simulink model "test2"  (R2022b)
settings: Solver=VariableStepAuto  StartTime=0.0  StopTime=30.0  RelTol=1e-3
undefined symbols (not defined in the file): fdesignblkfcn, gcbh
libraries: dspfdesign x4, vrlib x1
settings Model: Creator=elsibo  LastModifiedBy=ankurkohli007
settings DebuggingCC: UnconnectedInputMsg=warning  UnconnectedOutputMsg=warning  UnconnectedLineMsg=warning
settings ModelReferenceCC: EnableRefExpFcnMdlSchedulingChecks=on
settings RTWCC: DLArmComputeVersion=19.05

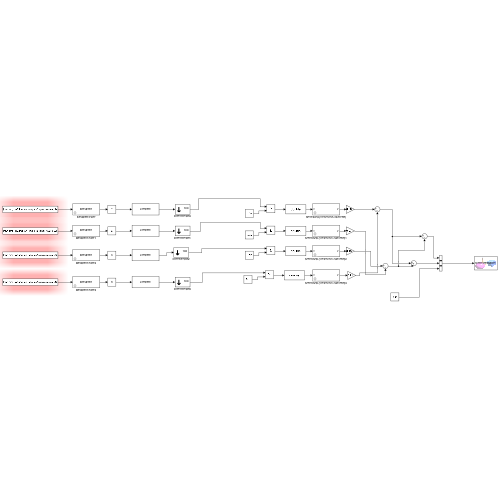
[thumbnail: Simulink's stored preview of the top-level diagram]
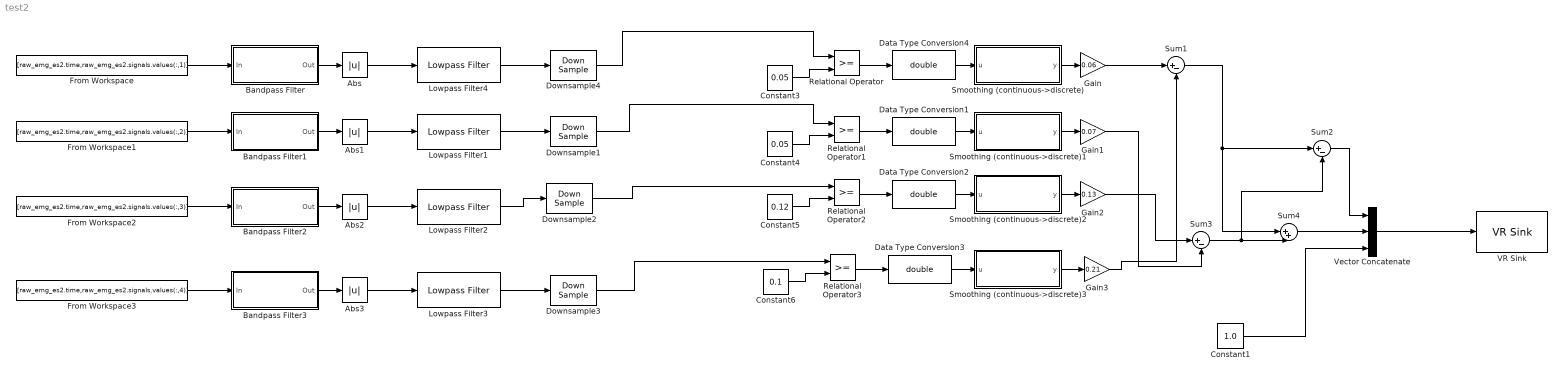
== system test2 ==
  Abs{,1..3} (4 alike) : Abs  SaturateOnIntegerOverflow=off
  Bandpass Filter : Subsystem  DialogController=fdesignblkfcn  InitFcn=fdesignblkfcn(gcbh, {'InitFcn'});  mask(Bandpass Filter){}
      mask help: Design a bandpass filter
      settings: CopyFcn=fdesignblkfcn(gcbh, {'CopyFcn'});
      mask Help: helpview(mapfilelocation('dsp'), 'dspbandpassfilter');
      mask Display: disp('Bandpass');
  Bandpass Filter1 : Subsystem  DialogController=fdesignblkfcn  InitFcn=fdesignblkfcn(gcbh, {'InitFcn'});  mask(Bandpass Filter){}
      mask help: Design a bandpass filter
      settings: CopyFcn=fdesignblkfcn(gcbh, {'CopyFcn'});
      mask Help: helpview(mapfilelocation('dsp'), 'dspbandpassfilter');
      mask Display: disp('Bandpass');
  Bandpass Filter2 : Subsystem  DialogController=fdesignblkfcn  InitFcn=fdesignblkfcn(gcbh, {'InitFcn'});  mask(Bandpass Filter){}
      mask help: Design a bandpass filter
      settings: CopyFcn=fdesignblkfcn(gcbh, {'CopyFcn'});
      mask Help: helpview(mapfilelocation('dsp'), 'dspbandpassfilter');
      mask Display: disp('Bandpass');
  Bandpass Filter3 : Subsystem  DialogController=fdesignblkfcn  InitFcn=fdesignblkfcn(gcbh, {'InitFcn'});  mask(Bandpass Filter){}
      mask help: Design a bandpass filter
      settings: CopyFcn=fdesignblkfcn(gcbh, {'CopyFcn'});
      mask Help: helpview(mapfilelocation('dsp'), 'dspbandpassfilter');
      mask Display: disp('Bandpass');
  Constant1 : Constant  Value=1.0
  Constant3 : Constant  Value=0.05
  Constant4 : Constant  Value=0.05
  Constant5 : Constant  Value=0.12
  Constant6 : Constant  Value=0.1
  Data Type Conversion{1..4} (4 alike) : DataTypeConversion  OutMin=[0.2]  OutMax=[1000]  OutDataTypeStr=double  SaturateOnIntegerOverflow=off  RndMeth=Floor
  Downsample{1..4} (4 alike) : DownSample  N=100  RateOptions=Allow multirate processing
  From Workspace : FromWorkspace  VariableName=[raw_emg_es2.time,raw_emg_es2.signals.values(:,1)]  SampleTime=1/3000
  From Workspace1 : FromWorkspace  VariableName=[raw_emg_es2.time,raw_emg_es2.signals.values(:,2)]  SampleTime=1/3000
  From Workspace2 : FromWorkspace  VariableName=[raw_emg_es2.time,raw_emg_es2.signals.values(:,3)]  SampleTime=1/3000
  From Workspace3 : FromWorkspace  VariableName=[raw_emg_es2.time,raw_emg_es2.signals.values(:,4)]  SampleTime=1/3000
  Gain : Gain  Gain=0.06
  Gain1 : Gain  Gain=0.07
  Gain2 : Gain  Gain=0.13
  Gain3 : Gain  Gain=0.21
  Lowpass Filter{1..4} (4 alike) : dspfdesign/Lowpass Filter  FilterType=FIR  DesignForMinimumOrder=on  FilterOrder=50  PassbandFrequency=3e3  StopbandFrequency=5e3  PassbandRipple=0.1  StopbandAttenuation=80  InheritSampleRate=off  SampleRate=44100  SimulateUsing=Interpreted execution  roundingMode=Floor  coeffsDataTypeStr=fixdt(1,16)
  Relational Operator{,1..3} (4 alike) : RelationalOperator  OutDataTypeStr=boolean  RndMeth=Simplest  InputSameDT=off
  Smoothing (continuous->discrete) : Subsystem  mask(Smoothing (continuous->discrete)){tsSmoothing=0.35, smoothing0=0}
      mask prompts: tsSmoothing "physmod:simscape:couplers:SimscapeNetworkCouplersLib:SmoothingTimeConstants_MP"; smoothing0 "physmod:simscape:couplers:SimscapeNetworkCouplersLib:InitialOutput_MP"
      mask help: physmod:simscape:couplers:SimscapeNetworkCouplersLib:Smoothingcontinuousdiscrete_MD
      mask Help: web([docroot '/physmod/simscape/ref/networkcouplersmoothingcontinuousdiscrete.html'])
  Smoothing (continuous->discrete)1 : Subsystem  mask(Smoothing (continuous->discrete)){tsSmoothing=0.35, smoothing0=0}
      mask prompts: tsSmoothing "physmod:simscape:couplers:SimscapeNetworkCouplersLib:SmoothingTimeConstants_MP"; smoothing0 "physmod:simscape:couplers:SimscapeNetworkCouplersLib:InitialOutput_MP"
      mask help: physmod:simscape:couplers:SimscapeNetworkCouplersLib:Smoothingcontinuousdiscrete_MD
      mask Help: web([docroot '/physmod/simscape/ref/networkcouplersmoothingcontinuousdiscrete.html'])
  Smoothing (continuous->discrete)2 : Subsystem  mask(Smoothing (continuous->discrete)){tsSmoothing=0.35, smoothing0=0}
      mask prompts: tsSmoothing "physmod:simscape:couplers:SimscapeNetworkCouplersLib:SmoothingTimeConstants_MP"; smoothing0 "physmod:simscape:couplers:SimscapeNetworkCouplersLib:InitialOutput_MP"
      mask help: physmod:simscape:couplers:SimscapeNetworkCouplersLib:Smoothingcontinuousdiscrete_MD
      mask Help: web([docroot '/physmod/simscape/ref/networkcouplersmoothingcontinuousdiscrete.html'])
  Smoothing (continuous->discrete)3 : Subsystem  mask(Smoothing (continuous->discrete)){tsSmoothing=0.35, smoothing0=0}
      mask prompts: tsSmoothing "physmod:simscape:couplers:SimscapeNetworkCouplersLib:SmoothingTimeConstants_MP"; smoothing0 "physmod:simscape:couplers:SimscapeNetworkCouplersLib:InitialOutput_MP"
      mask help: physmod:simscape:couplers:SimscapeNetworkCouplersLib:Smoothingcontinuousdiscrete_MD
      mask Help: web([docroot '/physmod/simscape/ref/networkcouplersmoothingcontinuousdiscrete.html'])
  Sum1 : Sum  Inputs=|+-
  Sum2 : Sum  Inputs=|+-
  Sum3 : Sum  Inputs=|+-
  Sum4 : Sum  Inputs=|++
  VR Sink : vrlib/VR Sink  InstantiateOnLoad=on  SampleTime=0.1  ViewEnable=on  RemoteChange=off  RemoteView=off  FieldsWritten=cursor.translation.3.1.1.double  WorldFileName=8_palline_color.wrl  AutoView=off  VideoDimensions=[]  AllowVariableSize=off
  Vector Concatenate : Concatenate  NumInputs=3
  wires:
  From Workspace/1 -> Bandpass Filter/1(In)
  Bandpass Filter/1(Out) -> Abs/1
  Abs/1 -> Lowpass Filter4/1
  Lowpass Filter4/1 -> Downsample4/1
  Abs1/1 -> Lowpass Filter1/1
  Lowpass Filter1/1 -> Downsample1/1
  Bandpass Filter1/1(Out) -> Abs1/1
  From Workspace1/1 -> Bandpass Filter1/1(In)
  Downsample1/1 -> Relational Operator1/1
  Abs2/1 -> Lowpass Filter2/1
  Bandpass Filter2/1(Out) -> Abs2/1
  From Workspace2/1 -> Bandpass Filter2/1(In)
  Downsample2/1 -> Relational Operator2/1
  Abs3/1 -> Lowpass Filter3/1
  Lowpass Filter3/1 -> Downsample3/1
  Bandpass Filter3/1(Out) -> Abs3/1
  From Workspace3/1 -> Bandpass Filter3/1(In)
  Downsample3/1 -> Relational Operator3/1
  Vector Concatenate/1 -> VR Sink/1
  Downsample4/1 -> Relational Operator/1
  Constant3/1 -> Relational Operator/2
  Relational Operator/1 -> Data Type Conversion4/1
  Relational Operator1/1 -> Data Type Conversion1/1
  Constant4/1 -> Relational Operator1/2
  Relational Operator2/1 -> Data Type Conversion2/1
  Constant5/1 -> Relational Operator2/2
  Relational Operator3/1 -> Data Type Conversion3/1
  Constant6/1 -> Relational Operator3/2
  Lowpass Filter2/1 -> Downsample2/1
  Data Type Conversion3/1 -> Smoothing (continuous->discrete)3/1(u)
  Data Type Conversion2/1 -> Smoothing (continuous->discrete)2/1(u)
  Data Type Conversion1/1 -> Smoothing (continuous->discrete)1/1(u)
  Data Type Conversion4/1 -> Smoothing (continuous->discrete)/1(u)
  Smoothing (continuous->discrete)/1(y) -> Gain/1
  Smoothing (continuous->discrete)1/1(y) -> Gain1/1
  Smoothing (continuous->discrete)2/1(y) -> Gain2/1
  Smoothing (continuous->discrete)3/1(y) -> Gain3/1
  Gain/1 -> Sum1/1
  Sum1/1 -> Sum2/1, Sum4/1
  Gain2/1 -> Sum3/1
  Sum3/1 -> Sum4/2, Sum2/2
  Sum4/1 -> Vector Concatenate/2
  Sum2/1 -> Vector Concatenate/1
  Constant1/1 -> Vector Concatenate/3
  Gain3/1 -> Sum1/2
  Gain1/1 -> Sum3/2

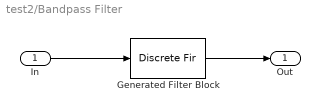
== system test2/Bandpass Filter ==
  In : Inport
  Generated Filter Block : DiscreteFir  Tag=BlockMethodSubSystem  Coefficients=[-0.0867106986736685681 0.172879501957226178 0.0611368344740756825 0.00822498172698654662 -0.0189364689630777752 -0.0305456119635362962 -0.029927052061019966 -0.0224311445482471734 -0.0154422453333472702 -0.0147705811987406625 -0.0205783857487597949 -0.0272517797256104505 -0.0284569945610830509 -0.0221839585574007091 -0.0127406715665240016 -0.00735000555653291324 -0.0102169041814385748 -0.0189181160821402621 -0.0260072397446443268 -0.0250951422264934776 -0.0162958899444141936 -0.00644643769533894805 -0.00372657608997871599 -0.0107951272745376546 -0.0221929620414225356 -0.0284553825598440994 -0.0237986889434766841 -0.0113779247022730377 -0.00119952503274776186 -0.00224663464687881349 -0.0146779403633768464 -0.0289282353463493902 -0.0329178478450258896 -0.0221510441115707439 -0.00434610570060027946 0.00573186727481306366 -0.00179813231379483346 -0.023001586974820111 -0.0413251082228547201 -0.0401288838953623231 -0.0168514574192910466 0.0121051446615590193 0.0218215231144973931 -0.00171807992762008032 -0.0470242140764826691 -0.0802559080529268998 -0.0639028947733619318 0.0153185042045271922 0.13460237441843137 0.241443784310572063 0.283829886850723301 0.241443784310572063 0.13460237441843137 0.0153185042045271922 -0.0639028947733619318 -0.0802559080529268998 -0.0470242140764826691 -0.00171807992762008032 0.0218215231144973931 0.0121051446615590193 -0.0168514574192910466 -0.0401288838953623231 -0.0413251082228547201 -0.023001586974820111 -0.00179813231379483346 0.00573186727481306366 -0.00434610570060027946 -0.0221510441115707439 -0.0329178478450258896 -0.0289282353463493902 -0.0146779403633768464 -0.00224663464687881349 -0.00119952503274776186 -0.0113779247022730377 -0.0237986889434766841 -0.0284553825598440994 -0.0221929620414225356 -0.0107951272745376546 -0.00372657608997871599 -0.00644643769533894805 -0.0162958899444141936 -0.0250951422264934776 -0.0260072397446443268 -0.0189181160821402621 -0.0102169041814385748 -0.00735000555653291324 -0.0127406715665240016 -0.0221839585574007091 -0.0284569945610830509 -0.0272517797256104505 -0.0205783857487597949 -0.0147705811987406625 -0.0154422453333472702 -0.0224311445482471734 -0.029927052061019966 -0.0305456119635362962 -0.0189364689630777752 0.00822498172698654662 0.0611368344740756825 0.172879501957226178 -0.0867106986736685681]  InputProcessing=Columns as channels (frame based)
  Out : Outport  VectorParamsAs1DForOutWhenUnconnected=off
  wires:
  In/1 -> Generated Filter Block/1
  Generated Filter Block/1 -> Out/1

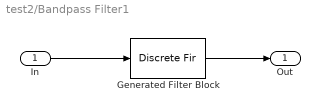
== system test2/Bandpass Filter1 ==
  In : Inport
  Generated Filter Block : DiscreteFir  Tag=BlockMethodSubSystem  Coefficients=[-0.0867106986736685681 0.172879501957226178 0.0611368344740756825 0.00822498172698654662 -0.0189364689630777752 -0.0305456119635362962 -0.029927052061019966 -0.0224311445482471734 -0.0154422453333472702 -0.0147705811987406625 -0.0205783857487597949 -0.0272517797256104505 -0.0284569945610830509 -0.0221839585574007091 -0.0127406715665240016 -0.00735000555653291324 -0.0102169041814385748 -0.0189181160821402621 -0.0260072397446443268 -0.0250951422264934776 -0.0162958899444141936 -0.00644643769533894805 -0.00372657608997871599 -0.0107951272745376546 -0.0221929620414225356 -0.0284553825598440994 -0.0237986889434766841 -0.0113779247022730377 -0.00119952503274776186 -0.00224663464687881349 -0.0146779403633768464 -0.0289282353463493902 -0.0329178478450258896 -0.0221510441115707439 -0.00434610570060027946 0.00573186727481306366 -0.00179813231379483346 -0.023001586974820111 -0.0413251082228547201 -0.0401288838953623231 -0.0168514574192910466 0.0121051446615590193 0.0218215231144973931 -0.00171807992762008032 -0.0470242140764826691 -0.0802559080529268998 -0.0639028947733619318 0.0153185042045271922 0.13460237441843137 0.241443784310572063 0.283829886850723301 0.241443784310572063 0.13460237441843137 0.0153185042045271922 -0.0639028947733619318 -0.0802559080529268998 -0.0470242140764826691 -0.00171807992762008032 0.0218215231144973931 0.0121051446615590193 -0.0168514574192910466 -0.0401288838953623231 -0.0413251082228547201 -0.023001586974820111 -0.00179813231379483346 0.00573186727481306366 -0.00434610570060027946 -0.0221510441115707439 -0.0329178478450258896 -0.0289282353463493902 -0.0146779403633768464 -0.00224663464687881349 -0.00119952503274776186 -0.0113779247022730377 -0.0237986889434766841 -0.0284553825598440994 -0.0221929620414225356 -0.0107951272745376546 -0.00372657608997871599 -0.00644643769533894805 -0.0162958899444141936 -0.0250951422264934776 -0.0260072397446443268 -0.0189181160821402621 -0.0102169041814385748 -0.00735000555653291324 -0.0127406715665240016 -0.0221839585574007091 -0.0284569945610830509 -0.0272517797256104505 -0.0205783857487597949 -0.0147705811987406625 -0.0154422453333472702 -0.0224311445482471734 -0.029927052061019966 -0.0305456119635362962 -0.0189364689630777752 0.00822498172698654662 0.0611368344740756825 0.172879501957226178 -0.0867106986736685681]  InputProcessing=Columns as channels (frame based)
  Out : Outport  VectorParamsAs1DForOutWhenUnconnected=off
  wires:
  In/1 -> Generated Filter Block/1
  Generated Filter Block/1 -> Out/1

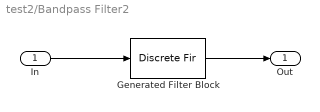
== system test2/Bandpass Filter2 ==
  In : Inport
  Generated Filter Block : DiscreteFir  Tag=BlockMethodSubSystem  Coefficients=[-0.0867106986736685681 0.172879501957226178 0.0611368344740756825 0.00822498172698654662 -0.0189364689630777752 -0.0305456119635362962 -0.029927052061019966 -0.0224311445482471734 -0.0154422453333472702 -0.0147705811987406625 -0.0205783857487597949 -0.0272517797256104505 -0.0284569945610830509 -0.0221839585574007091 -0.0127406715665240016 -0.00735000555653291324 -0.0102169041814385748 -0.0189181160821402621 -0.0260072397446443268 -0.0250951422264934776 -0.0162958899444141936 -0.00644643769533894805 -0.00372657608997871599 -0.0107951272745376546 -0.0221929620414225356 -0.0284553825598440994 -0.0237986889434766841 -0.0113779247022730377 -0.00119952503274776186 -0.00224663464687881349 -0.0146779403633768464 -0.0289282353463493902 -0.0329178478450258896 -0.0221510441115707439 -0.00434610570060027946 0.00573186727481306366 -0.00179813231379483346 -0.023001586974820111 -0.0413251082228547201 -0.0401288838953623231 -0.0168514574192910466 0.0121051446615590193 0.0218215231144973931 -0.00171807992762008032 -0.0470242140764826691 -0.0802559080529268998 -0.0639028947733619318 0.0153185042045271922 0.13460237441843137 0.241443784310572063 0.283829886850723301 0.241443784310572063 0.13460237441843137 0.0153185042045271922 -0.0639028947733619318 -0.0802559080529268998 -0.0470242140764826691 -0.00171807992762008032 0.0218215231144973931 0.0121051446615590193 -0.0168514574192910466 -0.0401288838953623231 -0.0413251082228547201 -0.023001586974820111 -0.00179813231379483346 0.00573186727481306366 -0.00434610570060027946 -0.0221510441115707439 -0.0329178478450258896 -0.0289282353463493902 -0.0146779403633768464 -0.00224663464687881349 -0.00119952503274776186 -0.0113779247022730377 -0.0237986889434766841 -0.0284553825598440994 -0.0221929620414225356 -0.0107951272745376546 -0.00372657608997871599 -0.00644643769533894805 -0.0162958899444141936 -0.0250951422264934776 -0.0260072397446443268 -0.0189181160821402621 -0.0102169041814385748 -0.00735000555653291324 -0.0127406715665240016 -0.0221839585574007091 -0.0284569945610830509 -0.0272517797256104505 -0.0205783857487597949 -0.0147705811987406625 -0.0154422453333472702 -0.0224311445482471734 -0.029927052061019966 -0.0305456119635362962 -0.0189364689630777752 0.00822498172698654662 0.0611368344740756825 0.172879501957226178 -0.0867106986736685681]  InputProcessing=Columns as channels (frame based)
  Out : Outport  VectorParamsAs1DForOutWhenUnconnected=off
  wires:
  In/1 -> Generated Filter Block/1
  Generated Filter Block/1 -> Out/1

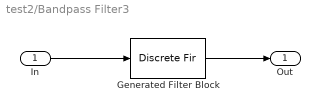
== system test2/Bandpass Filter3 ==
  In : Inport
  Generated Filter Block : DiscreteFir  Tag=BlockMethodSubSystem  Coefficients=[-0.0867106986736685681 0.172879501957226178 0.0611368344740756825 0.00822498172698654662 -0.0189364689630777752 -0.0305456119635362962 -0.029927052061019966 -0.0224311445482471734 -0.0154422453333472702 -0.0147705811987406625 -0.0205783857487597949 -0.0272517797256104505 -0.0284569945610830509 -0.0221839585574007091 -0.0127406715665240016 -0.00735000555653291324 -0.0102169041814385748 -0.0189181160821402621 -0.0260072397446443268 -0.0250951422264934776 -0.0162958899444141936 -0.00644643769533894805 -0.00372657608997871599 -0.0107951272745376546 -0.0221929620414225356 -0.0284553825598440994 -0.0237986889434766841 -0.0113779247022730377 -0.00119952503274776186 -0.00224663464687881349 -0.0146779403633768464 -0.0289282353463493902 -0.0329178478450258896 -0.0221510441115707439 -0.00434610570060027946 0.00573186727481306366 -0.00179813231379483346 -0.023001586974820111 -0.0413251082228547201 -0.0401288838953623231 -0.0168514574192910466 0.0121051446615590193 0.0218215231144973931 -0.00171807992762008032 -0.0470242140764826691 -0.0802559080529268998 -0.0639028947733619318 0.0153185042045271922 0.13460237441843137 0.241443784310572063 0.283829886850723301 0.241443784310572063 0.13460237441843137 0.0153185042045271922 -0.0639028947733619318 -0.0802559080529268998 -0.0470242140764826691 -0.00171807992762008032 0.0218215231144973931 0.0121051446615590193 -0.0168514574192910466 -0.0401288838953623231 -0.0413251082228547201 -0.023001586974820111 -0.00179813231379483346 0.00573186727481306366 -0.00434610570060027946 -0.0221510441115707439 -0.0329178478450258896 -0.0289282353463493902 -0.0146779403633768464 -0.00224663464687881349 -0.00119952503274776186 -0.0113779247022730377 -0.0237986889434766841 -0.0284553825598440994 -0.0221929620414225356 -0.0107951272745376546 -0.00372657608997871599 -0.00644643769533894805 -0.0162958899444141936 -0.0250951422264934776 -0.0260072397446443268 -0.0189181160821402621 -0.0102169041814385748 -0.00735000555653291324 -0.0127406715665240016 -0.0221839585574007091 -0.0284569945610830509 -0.0272517797256104505 -0.0205783857487597949 -0.0147705811987406625 -0.0154422453333472702 -0.0224311445482471734 -0.029927052061019966 -0.0305456119635362962 -0.0189364689630777752 0.00822498172698654662 0.0611368344740756825 0.172879501957226178 -0.0867106986736685681]  InputProcessing=Columns as channels (frame based)
  Out : Outport  VectorParamsAs1DForOutWhenUnconnected=off
  wires:
  In/1 -> Generated Filter Block/1
  Generated Filter Block/1 -> Out/1

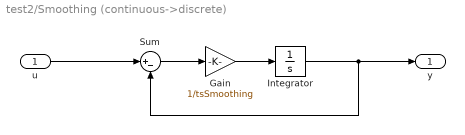
== system test2/Smoothing (continuous->discrete) ==
  u : Inport
  Gain : Gain  Gain=1/tsSmoothing
  Integrator : Integrator  InitialCondition=smoothing0
  Sum : Sum  Inputs=|+-
  y : Outport
  wires:
  u/1 -> Sum/1
  Integrator/1 -> Sum/2, y/1
  Gain/1 -> Integrator/1
  Sum/1 -> Gain/1

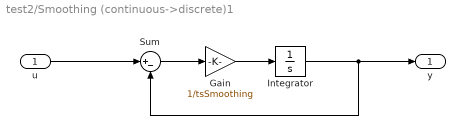
== system test2/Smoothing (continuous->discrete)1 ==
  u : Inport
  Gain : Gain  Gain=1/tsSmoothing
  Integrator : Integrator  InitialCondition=smoothing0
  Sum : Sum  Inputs=|+-
  y : Outport
  wires:
  u/1 -> Sum/1
  Integrator/1 -> Sum/2, y/1
  Gain/1 -> Integrator/1
  Sum/1 -> Gain/1

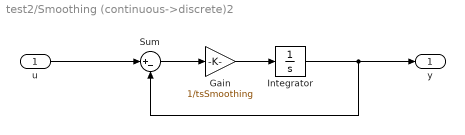
== system test2/Smoothing (continuous->discrete)2 ==
  u : Inport
  Gain : Gain  Gain=1/tsSmoothing
  Integrator : Integrator  InitialCondition=smoothing0
  Sum : Sum  Inputs=|+-
  y : Outport
  wires:
  u/1 -> Sum/1
  Integrator/1 -> Sum/2, y/1
  Gain/1 -> Integrator/1
  Sum/1 -> Gain/1

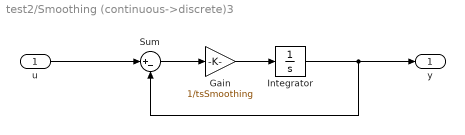
== system test2/Smoothing (continuous->discrete)3 ==
  u : Inport
  Gain : Gain  Gain=1/tsSmoothing
  Integrator : Integrator  InitialCondition=smoothing0
  Sum : Sum  Inputs=|+-
  y : Outport
  wires:
  u/1 -> Sum/1
  Integrator/1 -> Sum/2, y/1
  Gain/1 -> Integrator/1
  Sum/1 -> Gain/1
